simulink model "RES_lab2"  (R2020b)
settings: Solver=VariableStepAuto  StartTime=0.0  StopTime=10.0  RelTol=1e-3
libraries: powerlib x22, simulink x2
settings Model: Creator=Lenovo  LastModifiedBy=Priya
settings DebuggingCC: AlgebraicLoopMsg=none

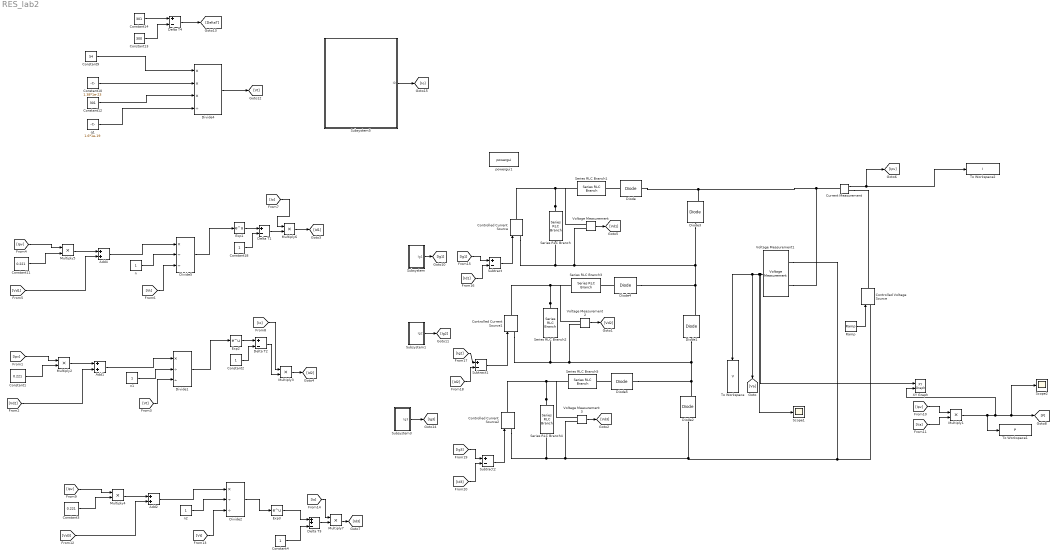
== system RES_lab2 ==
  Add1 : Sum
  Add2 : Sum
  Add4 : Sum
  Constant1 : Constant  Value=0.221
  Constant10 : Constant  Value=1.38*1e-23
  Constant11 : Constant  Value=0.221
  Constant12 : Constant  Value=301
  Constant13 : Constant  Value=300
  Constant14 : Constant  Value=301
  Constant18 : Constant
  Constant2 : Constant
  Constant3 : Constant  Value=0.221
  Constant4 : Constant
  Constant9 : Constant  Value=54
  Controlled Current Source : powerlib/Electrical Sources/Controlled Current Source  Initialize=on  Source_Type=AC  Amplitude=0  Phase=0  Frequency=0  Measurements=None
  Controlled Current Source1 : powerlib/Electrical Sources/Controlled Current Source  Initialize=on  Source_Type=AC  Amplitude=0  Phase=0  Frequency=0  Measurements=None
  Controlled Current Source2 : powerlib/Electrical Sources/Controlled Current Source  Initialize=on  Source_Type=AC  Amplitude=0  Phase=0  Frequency=0  Measurements=None
  Controlled Voltage Source : powerlib/Electrical Sources/Controlled Voltage Source  Initialize=on  Source_Type=AC  Amplitude=0  Phase=0  Frequency=0  Measurements=None
  Current Measurement : powerlib/Measurements/Current Measurement  PhasorSimulation=off  OutputType=Complex  PSBequivalent=0
  Delta T1 : Sum  Inputs=+-
  Delta T2 : Sum  Inputs=+-
  Delta T3 : Sum  Inputs=++-
  Delta T4 : Sum  Inputs=+-
  Diode : powerlib/Power Electronics/Diode  Ron=0.001  Lon=0  Vf=0.8  IC=0  UseSnubber=0  Rs=500  Cs=250e-9  Measurements=off
  Diode1 : powerlib/Power Electronics/Diode  Ron=0.001  Lon=0  Vf=0.8  IC=0  UseSnubber=0  Rs=0  Cs=0  Measurements=on
  Diode2 : powerlib/Power Electronics/Diode  Ron=0.001  Lon=0  Vf=0.8  IC=0  UseSnubber=0  Rs=0  Cs=0  Measurements=on
  Diode3 : powerlib/Power Electronics/Diode  Ron=0.001  Lon=0  Vf=0.8  IC=0  UseSnubber=0  Rs=0  Cs=0  Measurements=on
  Diode4 : powerlib/Power Electronics/Diode  Ron=0.001  Lon=0  Vf=0.8  IC=0  UseSnubber=0  Rs=500  Cs=250e-9  Measurements=off
  Diode5 : powerlib/Power Electronics/Diode  Ron=0.001  Lon=0  Vf=0.8  IC=0  UseSnubber=0  Rs=500  Cs=250e-9  Measurements=off
  Divide1 : Product  Inputs=*//
  Divide2 : Product  Inputs=*//
  Divide4 : Product  Inputs=***/
  Divide5 : Product  Inputs=*//
  Exp1 : Math  SignedPower=on  SaturateOnIntegerOverflow=on
  Exp2 : Math  SignedPower=on  SaturateOnIntegerOverflow=on
  Exp3 : Math  SignedPower=on  SaturateOnIntegerOverflow=on
  Multiply{1..7} (7 alike) : Product
  Ramp : simulink/Sources/Ramp  slope=100  start=0  InitialOutput=0
  Scope1 : Scope
  Scope2 : Scope
  Series RLC Branch : powerlib/Elements/Series RLC Branch  LConnTagsString=__new0  RConnTagsString=__new0  BranchType=R  Resistance=414.5  Inductance=1e-3  SetiL0=off  InitialCurrent=0  Capacitance=1e-6  Setx0=off  InitialVoltage=0  Measurements=None
  Series RLC Branch1 : powerlib/Elements/Series RLC Branch  LConnTagsString=__new0  RConnTagsString=__new0  BranchType=R  Resistance=0.221  Inductance=1e-3  SetiL0=off  InitialCurrent=0  Capacitance=1e-6  Setx0=off  InitialVoltage=0  Measurements=None
  Series RLC Branch2 : powerlib/Elements/Series RLC Branch  LConnTagsString=__new0  RConnTagsString=__new0  BranchType=R  Resistance=414.5  Inductance=1e-3  SetiL0=off  InitialCurrent=0  Capacitance=1e-6  Setx0=off  InitialVoltage=0  Measurements=None
  Series RLC Branch3 : powerlib/Elements/Series RLC Branch  LConnTagsString=__new0  RConnTagsString=__new0  BranchType=R  Resistance=0.221  Inductance=1e-3  SetiL0=off  InitialCurrent=0  Capacitance=1e-6  Setx0=off  InitialVoltage=0  Measurements=None
  Series RLC Branch4 : powerlib/Elements/Series RLC Branch  LConnTagsString=__new0  RConnTagsString=__new0  BranchType=R  Resistance=414.5  Inductance=1e-3  SetiL0=off  InitialCurrent=0  Capacitance=1e-6  Setx0=off  InitialVoltage=0  Measurements=None
  Series RLC Branch5 : powerlib/Elements/Series RLC Branch  LConnTagsString=__new0  RConnTagsString=__new0  BranchType=R  Resistance=0.221  Inductance=1e-3  SetiL0=off  InitialCurrent=0  Capacitance=1e-6  Setx0=off  InitialVoltage=0  Measurements=None
  Subsystem : Subsystem
  Subsystem1 : Subsystem
  Subsystem3 : Subsystem
  Subsystem5 : Subsystem
  Subtract : Sum  Inputs=+-
  Subtract1 : Sum  Inputs=+-
  Subtract2 : Sum  Inputs=+-
  To Workspace : ToWorkspace  VariableName=V  SampleTime=-1
  To Workspace1 : ToWorkspace  VariableName=P  SampleTime=-1
  To Workspace2 : ToWorkspace  VariableName=I  SampleTime=-1
  Voltage Measurement{,1..3} (4 alike) : powerlib/Measurements/Voltage Measurement  PhasorSimulation=off  OutputType=Complex  PSBequivalent=0
  XY Graph : simulink/Sinks/XY Graph  xmin=0  xmax=100  ymin=0  ymax=400  st=1
  n : Constant
  n1 : Constant
  n2 : Constant
  powergui1 : powerlib/powergui  Priority=1  SimulationMode=Continuous  SampleTime=50e-6  frequency=60  Iterations=50  frequencyindice=0  Pbase=100e6  ErrMax=1e-4  UnitsV=kV  UnitsW=MW  buscounter=0  FunctionMessages=off  echomessages=off  EnableUseOfTLC=off  CurrentSourceSwitches=off  DisableSnubberDevices=off  DisableRonSwitches=off  DisableVfSwitches=off  DisplayEquations=off  AutomaticDiscreteSolvers=off  SolverType=Tustin/Backward Euler (TBE)  Interpol=off  ExternalGateDelay=off  methode=off  Ts=100  x0status=blocks  SPID=on  SwTol=0  HookPort=off  NonlinearTolerance=1e-4  nMaxIteration=100  ContinueOnMaxIteration=off  RestoreLinks=warning  ResistiveCurrentMeasurement=off  Frange=[0:2:500]  Ylog=off  Xlog=on  ShowGrid=off  save=off  variable=ZData  structure=0  ZoomFFT=off  StartTime=0.0  cycles=1  DisplayStyle=1  fundamental=60  FreqAxis=off  MaxFrequency=1000  frequencyindicesteady=1  RmsSteady=1  display=off
  q1 : Constant  Value=1.6*1e-19
  wires:
  Ramp/1 -> Controlled Voltage Source/1
  [Va] -> Multiply1/2
  [Ipv] -> Multiply1/1
  Multiply1/1 -> To Workspace1/1, XY Graph/2, Scope2/1, [P]
  Current Measurement/1 -> To Workspace2/1, [Ipv]
  Voltage Measurement/1 -> [Vd1]
  Voltage Measurement2/1 -> [Vd2]
  Voltage Measurement3/1 -> [Vd3]
  Add4/1 -> Divide5/1
  [Vt] -> Divide5/3
  Constant11/1 -> Multiply5/2
  Constant18/1 -> Delta T1/2
  [Io] -> Multiply6/1
  Divide5/1 -> Exp1/1
  [Vd1] -> Add4/2
  Multiply6/1 -> [Id1]
  Multiply5/1 -> Add4/1
  Delta T1/1 -> Multiply6/2
  Exp1/1 -> Delta T1/1
  [Ipv] -> Multiply5/1
  n/1 -> Divide5/2
  Divide4/1 -> [Vt]
  Constant9/1 -> Divide4/1
  Delta T4/1 -> [DeltaT]
  Constant14/1 -> Delta T4/1
  q1/1 -> Divide4/4
  Constant13/1 -> Delta T4/2
  Constant10/1 -> Divide4/2
  Constant12/1 -> Divide4/3
  [Ig1] -> Subtract/1
  [Id1] -> Subtract/2
  Subtract/1 -> Controlled Current Source/1
  [Id2] -> Subtract1/2
  [Ig2] -> Subtract1/1
  Subtract1/1 -> Controlled Current Source1/1
  [Id3] -> Subtract2/2
  [Ig3] -> Subtract2/1
  Subtract2/1 -> Controlled Current Source2/1
  Voltage Measurement1/1 -> To Workspace/1, [Va], Scope1/1, XY Graph/1
  Multiply7/1 -> [Id3]
  Constant3/1 -> Multiply4/2
  Delta T3/1 -> Multiply7/2
  Exp3/1 -> Delta T3/1
  Divide2/1 -> Exp3/1
  Add2/1 -> Divide2/1
  Multiply4/1 -> Add2/1
  n2/1 -> Divide2/2
  [Io] -> Multiply7/1
  [Vt] -> Divide2/3
  Constant4/1 -> Delta T3/3
  [Ipv] -> Multiply4/1
  [Vd3] -> Add2/2
  Constant2/1 -> Delta T2/2
  [Io] -> Multiply3/1
  Add1/1 -> Divide1/1
  Exp2/1 -> Delta T2/1
  [Ipv] -> Multiply2/1
  [Vt] -> Divide1/3
  [Vd2] -> Add1/2
  Delta T2/1 -> Multiply3/2
  Multiply2/1 -> Add1/1
  Divide1/1 -> Exp2/1
  Multiply3/1 -> [Id2]
  Constant1/1 -> Multiply2/2
  n1/1 -> Divide1/2
  Subsystem/1(Ig1) -> [Ig1]
  Subsystem1/1(Ig2) -> [Ig2]
  Subsystem3/1(Ig3) -> [Ig3]
  Subsystem5/1(I0) -> [Io]
  connections:
  Voltage Measurement3/LConn2 -- Voltage Measurement1/LConn2 -- Controlled Voltage Source/LConn1 -- Diode2/LConn1 -- Controlled Current Source2/LConn1 -- Series RLC Branch4/RConn1
  Voltage Measurement2/LConn2 -- Diode5/RConn1 -- Diode2/RConn1 -- Diode1/LConn1 -- Controlled Current Source1/LConn1 -- Series RLC Branch2/RConn1
  Voltage Measurement/LConn2 -- Diode4/RConn1 -- Diode1/RConn1 -- Diode3/LConn1 -- Controlled Current Source/LConn1 -- Series RLC Branch/RConn1
  Current Measurement/RConn1 -- Controlled Voltage Source/RConn1
  Diode3/RConn1 -- Voltage Measurement1/LConn1 -- Current Measurement/LConn1 -- Diode/RConn1
  Series RLC Branch/LConn1 -- Series RLC Branch1/RConn1 -- Voltage Measurement/LConn1 -- Controlled Current Source/RConn1
  Diode/LConn1 -- Series RLC Branch1/LConn1
  Series RLC Branch2/LConn1 -- Series RLC Branch3/RConn1 -- Voltage Measurement2/LConn1 -- Controlled Current Source1/RConn1
  Diode4/LConn1 -- Series RLC Branch3/LConn1
  Series RLC Branch4/LConn1 -- Controlled Current Source2/RConn1 -- Series RLC Branch5/RConn1 -- Voltage Measurement3/LConn1
  Diode5/LConn1 -- Series RLC Branch5/LConn1

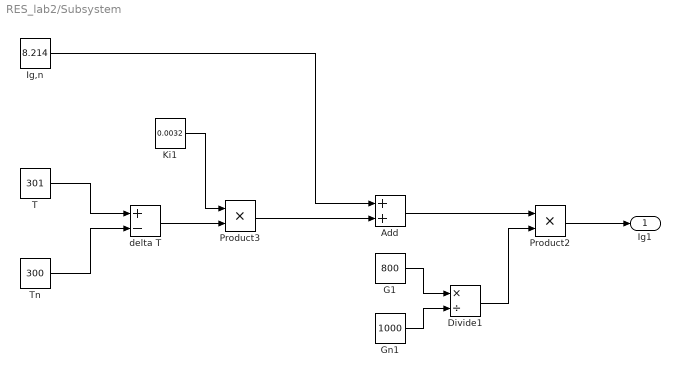
== system RES_lab2/Subsystem ==
  Add : Sum
  Divide1 : Product  Inputs=*/
  G1 : Constant  Value=800
  Gn1 : Constant  Value=1000
  Ig,n : Constant  Value=8.214
  Ki1 : Constant  Value=0.0032
  Product2 : Product
  Product3 : Product
  T : Constant  Value=301
  Tn : Constant  Value=300
  delta T : Sum  Inputs=+-
  Ig1 : Outport
  wires:
  Add/1 -> Product2/1
  Ig,n/1 -> Add/1
  Tn/1 -> delta T/2
  Gn1/1 -> Divide1/2
  T/1 -> delta T/1
  Product3/1 -> Add/2
  G1/1 -> Divide1/1
  Divide1/1 -> Product2/2
  delta T/1 -> Product3/2
  Ki1/1 -> Product3/1
  Product2/1 -> Ig1/1

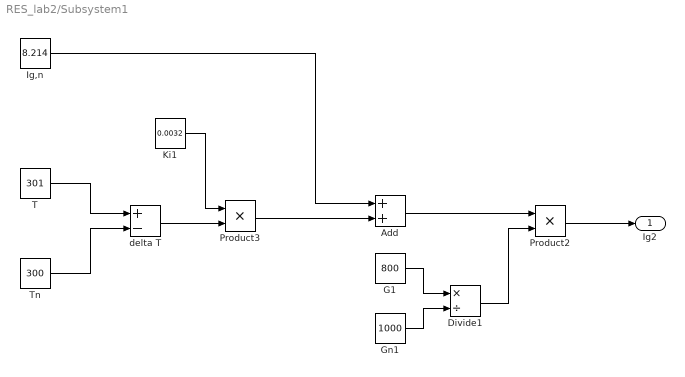
== system RES_lab2/Subsystem1 ==
  Add : Sum
  Divide1 : Product  Inputs=*/
  G1 : Constant  Value=800
  Gn1 : Constant  Value=1000
  Ig,n : Constant  Value=8.214
  Ki1 : Constant  Value=0.0032
  Product2 : Product
  Product3 : Product
  T : Constant  Value=301
  Tn : Constant  Value=300
  delta T : Sum  Inputs=+-
  Ig2 : Outport
  wires:
  Add/1 -> Product2/1
  Ig,n/1 -> Add/1
  Tn/1 -> delta T/2
  Gn1/1 -> Divide1/2
  T/1 -> delta T/1
  Product3/1 -> Add/2
  G1/1 -> Divide1/1
  Divide1/1 -> Product2/2
  delta T/1 -> Product3/2
  Ki1/1 -> Product3/1
  Product2/1 -> Ig2/1

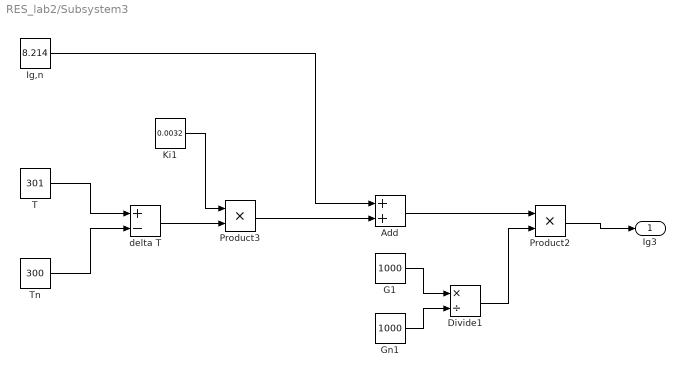
== system RES_lab2/Subsystem3 ==
  Add : Sum
  Divide1 : Product  Inputs=*/
  G1 : Constant  Value=1000
  Gn1 : Constant  Value=1000
  Ig,n : Constant  Value=8.214
  Ki1 : Constant  Value=0.0032
  Product2 : Product
  Product3 : Product
  T : Constant  Value=301
  Tn : Constant  Value=300
  delta T : Sum  Inputs=+-
  Ig3 : Outport
  wires:
  Add/1 -> Product2/1
  Ig,n/1 -> Add/1
  Tn/1 -> delta T/2
  Gn1/1 -> Divide1/2
  T/1 -> delta T/1
  Product3/1 -> Add/2
  G1/1 -> Divide1/1
  Divide1/1 -> Product2/2
  delta T/1 -> Product3/2
  Ki1/1 -> Product3/1
  Product2/1 -> Ig3/1

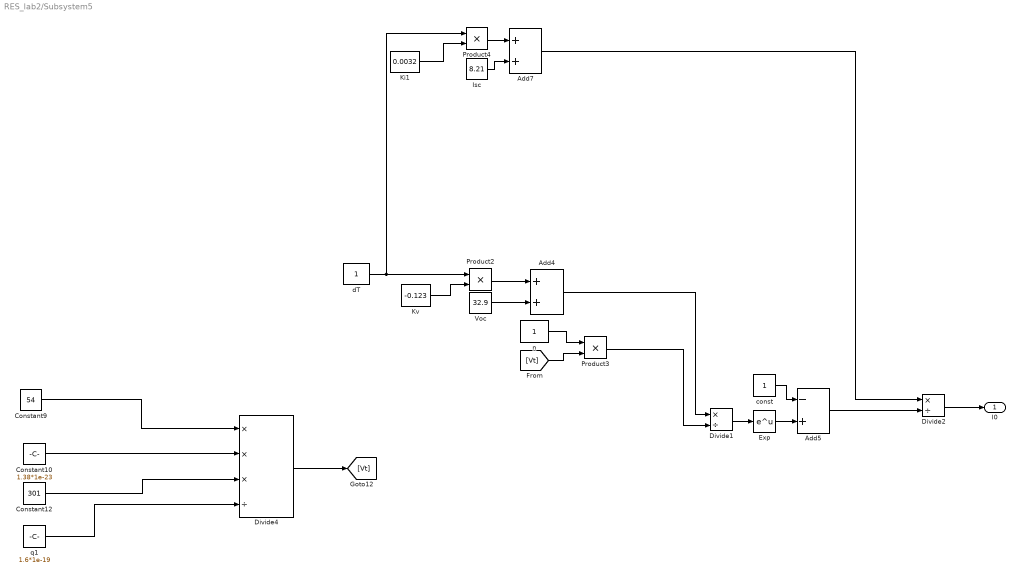
== system RES_lab2/Subsystem5 ==
  Add4 : Sum
  Add5 : Sum  Inputs=-+
  Add7 : Sum
  Constant10 : Constant  Value=1.38*1e-23
  Constant12 : Constant  Value=301
  Constant9 : Constant  Value=54
  Divide1 : Product  Inputs=*/
  Divide2 : Product  Inputs=*/
  Divide4 : Product  Inputs=***/
  Exp : Math  SaturateOnIntegerOverflow=on
  Isc : Constant  Value=8.21
  Ki1 : Constant  Value=0.0032
  Kv : Constant  Value=-0.123
  Product2 : Product
  Product3 : Product
  Product4 : Product
  Voc : Constant  Value=32.9
  const : Constant
  dT : Constant
  n : Constant
  q1 : Constant  Value=1.6*1e-19
  I0 : Outport
  wires:
  Constant9/1 -> Divide4/1
  [Vt] -> Product3/2
  Ki1/1 -> Product4/2
  Divide1/1 -> Exp/1
  q1/1 -> Divide4/4
  Divide4/1 -> [Vt]
  n/1 -> Product3/1
  Add5/1 -> Divide2/2
  Constant12/1 -> Divide4/3
  Product3/1 -> Divide1/2
  Add7/1 -> Divide2/1
  Isc/1 -> Add7/2
  dT/1 -> Product4/1, Product2/1
  Add4/1 -> Divide1/1
  Voc/1 -> Add4/2
  Divide2/1 -> I0/1
  const/1 -> Add5/1
  Exp/1 -> Add5/2
  Kv/1 -> Product2/2
  Product2/1 -> Add4/1
  Product4/1 -> Add7/1
  Constant10/1 -> Divide4/2
